simulink model "tarea1_retro"  (R2024a)
settings: Solver=VariableStepAuto  StartTime=0.0  StopTime=100  RelTol=1e-3

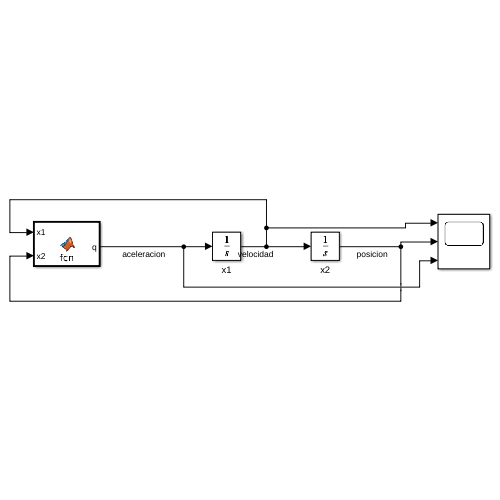
[thumbnail: Simulink's stored preview of the top-level diagram]
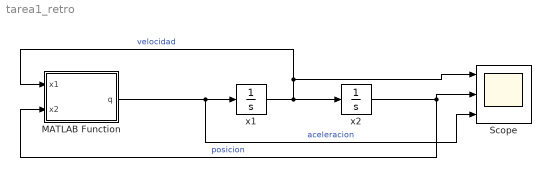
== system tarea1_retro ==
  MATLAB Function : MATLAB Function  TreatAsAtomicUnit=on
  Scope : Scope  NumInputPorts=3
  x1 : Integrator
  x2 : Integrator
  wires:
  x2/1 -> MATLAB Function/2(x2), Scope/2  "posicion"
  x1/1 -> x2/1, MATLAB Function/1(x1), Scope/1  "velocidad"
  MATLAB Function/1(q) -> Scope/3, x1/1  "aceleracion"

== matlab function tarea1_retro/MATLAB Function ==
  data: x1 input; x2 input; q output
function q = fcn(x1, x2)
k=.01;
m= 5;
l=.36;
g=9.8;
Tau=0;
a=l/2;
J=.75*m*(a*a);
q=(Tau-(m*g*a*cos(x2))-(k*x1))/J;
